simulink model "ident_HE"  (R2024b)
settings: Solver=FixedStepDiscrete  StartTime=0.0  StopTime=3500  FixedStep=1  RelTol=1e-3
libraries: slpidlib x1, pct23_lib x1
settings Model: Creator=MK  LastModifiedBy=patrik
settings DataIOCC: ReturnWorkspaceOutputs=off
settings OptimizationCC: ReuseModelBlockBuffer=off
settings DebuggingCC: UnconnectedInputMsg=warning  UnconnectedOutputMsg=warning  UnconnectedLineMsg=warning  ArithmeticOperatorsInVariantConditions=warning
settings ModelReferenceCC: EnableRefExpFcnMdlSchedulingChecks=on
settings SFSimCC: CustomCodeUndefinedFunction=UseInterfaceOnly
settings RTWCC: GPUComputeCapability=3.5  DLArmComputeVersion=19.05

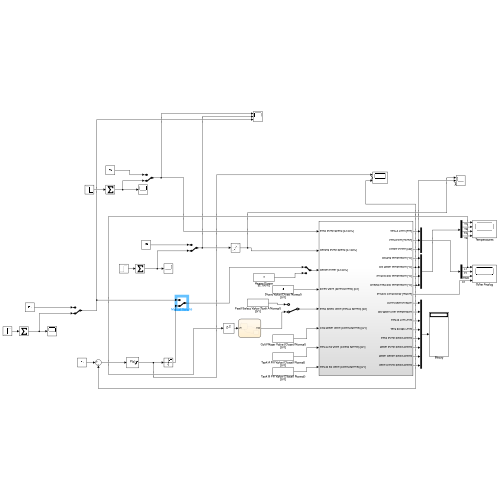
[thumbnail: Simulink's stored preview of the top-level diagram]
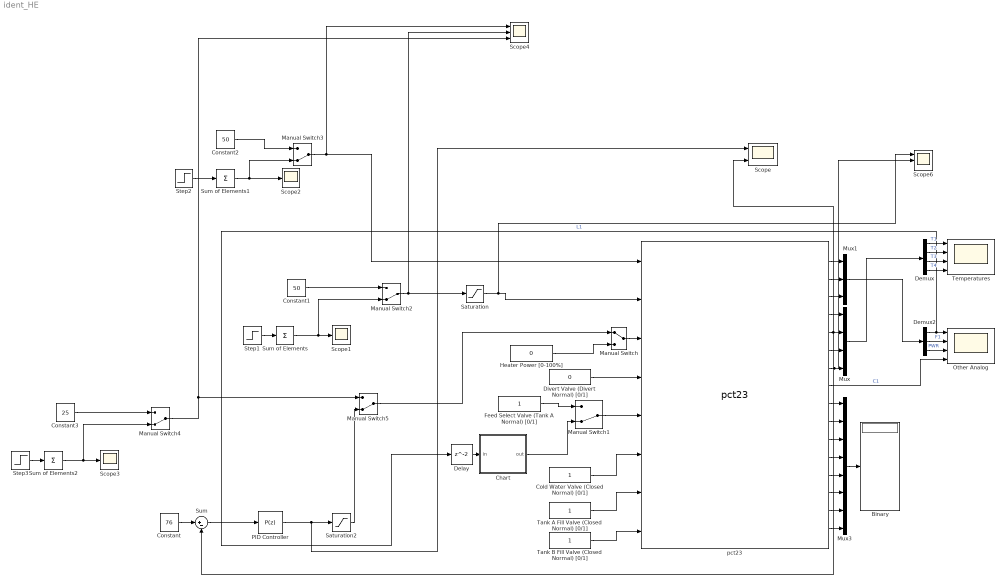
== system ident_HE ==
  Binary : Display
  Chart : Stateflow chart  TreatAsAtomicUnit=on
  Cold Water Valve (Closed Normal) [0/1] : Constant
  Constant : Constant  Value=76
  Constant1 : Constant  Value=50
  Constant2 : Constant  Value=50
  Constant3 : Constant  Value=25
  Delay : Delay
  Demux : Demux
  Demux2 : Demux  Outputs=3
  Divert Valve (Divert Normal) [0/1] : Constant  Value=0
  Feed Select Valve (Tank A Normal) [0/1] : Constant
  Heater Power [0-100%] : Constant  Value=0
  Manual Switch : ManualSwitch
  Manual Switch{1..5} (5 alike) : ManualSwitch  CurrentSetting=0
  Mux : Mux
  Mux1 : Mux  Inputs=3
  Mux3 : Mux  Inputs=8
  Other Analog : Scope  NumInputPorts=4
  PID Controller : slpidlib/PID Controller  Controller=P  Form=Ideal  TimeDomain=Discrete-time  UseExternalTs=off  SampleTime=-1  IntegratorMethod=Forward Euler  FilterMethod=Forward Euler  ControllerParametersSource=internal  P=12  I=10  UseKiTs=off  D=0  UseExternalDerivativeSource=off  N=100  UseFilter=on  TunerSelectOption=Transfer Function Based (PID Tuner App)  InitialConditionSource=internal  InitialConditionForIntegrator=0  InitialConditionForFilter=0  DifferentiatorICPrevScaledInput=0  ExternalReset=none  TrackingMode=off  Kt=1  LimitOutput=on  SatLimitsSource=internal  UpperSaturationLimit=100  LowerSaturationLimit=0  LinearizeAsGain=on  AntiWindupMode=clamping  Kb=1  LimitIntegrator=off  UpperIntegratorSaturationLimit=inf  LowerIntegratorSaturationLimit=-inf  POutMin=[]  POutMax=[]  IOutMin=[]  IOutMax=[]  DOutMin=[]  DOutMax=[]  NOutMin=[]  NOutMax=[]  SumOutMin=[]  SumOutMax=[]  SaturationOutMin=[]  SaturationOutMax=[]  PParamMin=[]  PParamMax=[]  IParamMin=[]  IParamMax=[]  DParamMin=[]  DParamMax=[]  NParamMin=[]  NParamMax=[]  KbParamMin=[]  KbParamMax=[]  KtParamMin=[]  KtParamMax=[]  KbOutMin=[]  KbOutMax=[]  KtOutMin=[]  KtOutMax=[]  IntegratorOutMin=[]  IntegratorOutMax=[]  FilterOutMin=[]  FilterOutMax=[]  SumI1OutMin=[]  SumI1OutMax=[]  SumI2OutMin=[]  SumI2OutMax=[]  SumI3OutMin=[]  SumI3OutMax=[]  SumI4OutMin=[]  SumI4OutMax=[]  SumDOutMin=[]  SumDOutMax=[]  DifferentiatorOutMin=[]  DifferentiatorOutMax=[]  FilterDiffOutCoefMin=[]  FilterDiffOutCoefMax=[]  ReciprocalOutMin=[]  ReciprocalOutMax=[]  SumDenOutMin=[]  SumDenOutMax=[]  SumNumOutMin=[]  SumNumOutMax=[]  DivideOutMin=[]  DivideOutMax=[]  UdiffTsProdOutMin=[]  UdiffTsProdOutMax=[]  NTsProdOutMin=[]  NTsProdOutMax=[]  UintegralTsProdOutMin=[]  UintegralTsProdOutMax=[]  UngainTsProdOutMin=[]  UngainTsProdOutMax=[]  ClampingZeroOutDataTypeStr=Inherit: Inherit via back propagation  ClampingZeroOutMin=[]  ClampingZeroOutMax=[]  FilterDenConstantOutDataTypeStr=Inherit: Inherit via back propagation  FilterDenConstantOutMin=[]  FilterDenConstantOutMax=[]  PCopyOutDataTypeStr=Inherit: Inherit via back propagation  PCopyOutMin=[]  PCopyOutMax=[]  NCopyOutDataTypeStr=Inherit: Inherit via back propagation  NCopyOutMin=[]  NCopyOutMax=[]  IntegratorContinuousStateAttributes=''  IntegratorStateMustResolveToSignalObject=off  IntegratorRTWStateStorageClass=Auto  FilterContinuousStateAttributes=''  FilterStateMustResolveToSignalObject=off  FilterRTWStateStorageClass=Auto  ParallelPVariant=InternalParameters  IdealPVariant=Disabled  IVariant=Disabled  DVariant=Disabled  IntegratorVariant=Disabled  SatVariant=Enabled  AWVariant=Disabled  PCopyVariant=Disabled  TRVariant=Disabled  FdbkBlocksVariant=Forward  IdealPFdbkVariant=Disabled  SatFdbkVariant=Disabled  DerivativeFilterVariant=Disabled  NVariant=Disabled  NCopyVariant=Disabled_SignalSpec  FilterICVariant=Disabled  IntegratorICVariant=Disabled  ExternalResetVariant=Disabled  TRSumVariant=Passthrough  SumFdbkVariant=Disabled  SumVariant=Passthrough_P  TsampFilterVariant=InternalTs  TsampNgainVariant=Passthrough  TsampIntegralVariant=Disabled_SignalSpec  ExternalSaturationOutDataTypeStr=Inherit: Same as second input  DerivativeSourceVariant=Disabled  PreIntVariant=InternalPreInt
  Saturation : Saturate  UpperLimit=100  LowerLimit=0
  Saturation2 : Saturate  UpperLimit=100  LowerLimit=0
  Scope : Scope  NumInputPorts=3
  Scope1 : Scope
  Scope2 : Scope
  Scope3 : Scope
  Scope4 : Scope  NumInputPorts=3
  Scope6 : Scope  NumInputPorts=3
  Step1 : Step  Time=[250, 500,750,1000,1250,1500,1750,2000,2250,2500,2750,3000,3250]  Before=[50, 0,0,0,0, 0,0,0,0, 0,0,0,0]  After=[100,-80,10,60,-40,20,-30,60,-80,30,20,-40,10]  SampleTime=0
  Step2 : Step  Time=[250, 500,750,1000,1250,1500,1750,2000,2250,2500,2750,3000,3250]  Before=[50, 0,0,0,0, 0,0,0,0, 0,0,0,0]  After=[30,80,-40,-30,50,-30,-10,60,-80,50,-40,60,-40]  SampleTime=0
  Step3 : Step  Time=[250, 500,750,1000,1250,1500,1750,2000,2250,2500,2750,3000,3250]  Before=[25, 0,0,0,0, 0,0,0,0, 0,0,0,0]  After=[25,-15,0,30,0,-15,0,-15,0,30,0,-15,0]  SampleTime=0
  Sum : Sum  Inputs=|+-
  Sum of Elements : Sum  Inputs=+
  Sum of Elements1 : Sum  Inputs=+
  Sum of Elements2 : Sum  Inputs=+
  Tank A Fill Valve (Closed Normal) [0/1] : Constant
  Tank B Fill Valve (Closed Normal) [0/1] : Constant
  Temperatures : Scope  NumInputPorts=4
  pct23 : pct23_lib/pct23  SystemSampleTime=-1  VariantActivationTime=update diagram  AllowFlexibleInterface=on  Latency=0  AutoFrameSizeCalculation=off
  wires:
  Manual Switch3/1 -> Scope4/1, pct23/1
  Tank B Fill Valve (Closed Normal) [0/1]/1 -> pct23/8
  Tank A Fill Valve (Closed Normal) [0/1]/1 -> pct23/7
  Cold Water Valve (Closed Normal) [0/1]/1 -> pct23/6
  Divert Valve (Divert Normal) [0/1]/1 -> pct23/4
  pct23/4 -> Mux/1
  pct23/5 -> Scope/3, Sum/2, Mux/2
  pct23/6 -> Mux/3
  Mux/1 -> Demux/1
  Demux/2 -> Temperatures/2  "T2"
  Demux/4 -> Temperatures/4  "T4"
  Demux/3 -> Temperatures/3  "T3"
  Demux/1 -> Temperatures/1  "T1"
  Demux2/1 -> Delay/1, Other Analog/1  "L1"
  Demux2/2 -> Other Analog/2  "F1"
  Demux2/3 -> Other Analog/3  "PWR"
  Mux1/1 -> Demux2/1
  pct23/8 -> Other Analog/4  "C1"
  pct23/1 -> Mux1/1
  pct23/2 -> Mux1/2
  pct23/3 -> Mux1/3
  Mux3/1 -> Binary/1
  pct23/9 -> Mux3/1
  pct23/10 -> Mux3/2
  pct23/11 -> Mux3/3
  pct23/12 -> Mux3/4
  pct23/13 -> Mux3/5
  pct23/14 -> Mux3/6
  pct23/15 -> Mux3/7
  pct23/16 -> Mux3/8
  Constant/1 -> Sum/1
  Sum/1 -> PID Controller/1
  PID Controller/1 -> Saturation2/1, Scope/1
  Heater Power [0-100%]/1 -> Manual Switch/2
  Manual Switch/1 -> pct23/3
  pct23/7 -> Scope6/2, Mux/4
  Saturation/1 -> Scope6/1, pct23/2
  Constant1/1 -> Manual Switch2/1
  Feed Select Valve (Tank A Normal) [0/1]/1 -> Manual Switch1/1
  Manual Switch1/1 -> pct23/5
  Chart/1(out) -> Manual Switch1/2
  Delay/1 -> Chart/1(in)
  Step1/1 -> Sum of Elements/1
  Sum of Elements/1 -> Scope1/1, Manual Switch2/2
  Sum of Elements1/1 -> Manual Switch3/2, Scope2/1
  Constant2/1 -> Manual Switch3/1
  Step2/1 -> Sum of Elements1/1
  Constant3/1 -> Manual Switch4/1
  Saturation2/1 -> Manual Switch5/2
  Manual Switch5/1 -> Manual Switch/1
  Manual Switch4/1 -> Scope4/3, Manual Switch5/1
  Step3/1 -> Sum of Elements2/1
  Sum of Elements2/1 -> Manual Switch4/2, Scope3/1
  Manual Switch2/1 -> Scope4/2, Saturation/1

== stateflow chart ident_HE/Chart ==
  state Close
    out = 1;
  state Open
    out = 0;
  (default) -> Close
  Close -> Open : [in<150]
  Open -> Close : [in>180]
  data: in input; out output
